simulink library "CPFSK_termpaper"  (R2018a)
settings: Solver=VariableStepAuto  StartTime=0.0  StopTime=10.0  RelTol=1e-3
libraries: dspfdesign x4, commchan3 x1, commrandsrc3 x1, commdigbbndcpm2 x1, simulink x1, dspswit3 x1
settings Model: Creator=Arun Sai  LastModifiedBy=Arun Sai

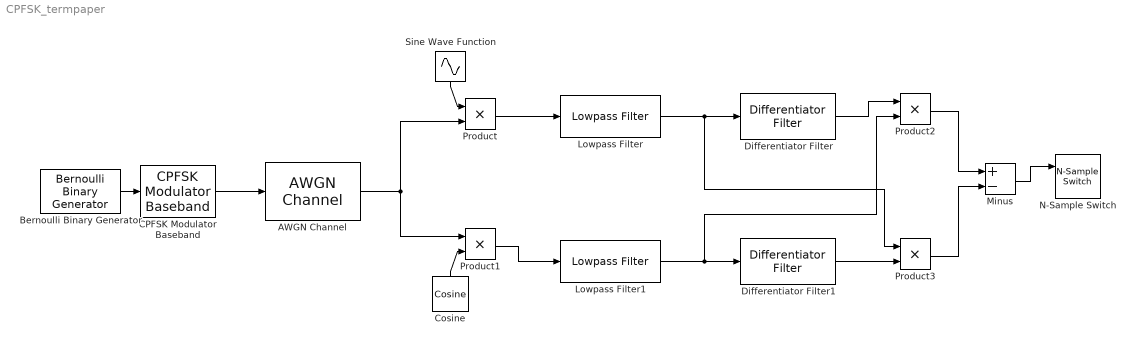
== system CPFSK_termpaper ==
  AWGN Channel : commchan3/AWGN Channel  InputProcessing=Columns as channels (frame based)  seed=67  noiseMode="Signal to noise ratio  (Eb/No)"  EbNodB=10  EsNodB=10  SNRdB=10  bitsPerSym=8  Ps=1  Tsym=1  variance=1
  Bernoulli Binary Generator : commrandsrc3/Bernoulli Binary Generator  ProbabilityOfZero=0.5  SeedSource=Auto  Seed=0  SampleTime=1  SamplesPerFrame=1  OutputDataType=double  SimulateUsing=Interpreted execution
  CPFSK Modulator Baseband : commdigbbndcpm2/CPFSK Modulator Baseband  Mnum=2  inputType=Integer  mappingType=Binary  modIdx=.67  phaseOffset=0  samplesPerSymbol=8  RateOptions=Enforce single-rate processing  outDataType=double
      settings: SourceProductName=Communications System Toolbox  SourceProductBaseCode=CM
  Cosine : simulink/Lookup Tables/Cosine  Formula=cos(2*pi*u)  NumDataPoints=(2^5)+1  OutputWordLength=16  InternalRulePriority=Speed
      settings: SourceProductName=Simulink  SourceProductBaseCode=SL
  Differentiator Filter : dspfdesign/Differentiator Filter  DesignForMinimumOrder=on  FilterOrder=31  PassbandRipple=0.1  ScaleCoefficients=off  SimulateUsing=Interpreted execution  roundingMode=Floor  coeffsDataTypeStr=fixdt(1,16)
      settings: SourceProductName=DSP System Toolbox  SourceProductBaseCode=DS
  Differentiator Filter1 : dspfdesign/Differentiator Filter  DesignForMinimumOrder=on  FilterOrder=31  PassbandRipple=0.1  ScaleCoefficients=off  SimulateUsing=Interpreted execution  roundingMode=Floor  coeffsDataTypeStr=fixdt(1,16)
      settings: SourceProductName=DSP System Toolbox  SourceProductBaseCode=DS
  Lowpass Filter : dspfdesign/Lowpass Filter  FilterType=FIR  DesignForMinimumOrder=on  FilterOrder=50  PassbandFrequency=8e3  StopbandFrequency=12e3  PassbandRipple=0.1  StopbandAttenuation=80  InheritSampleRate=off  SampleRate=44100  SimulateUsing=Interpreted execution  roundingMode=Floor  coeffsDataTypeStr=fixdt(1,16)
  Lowpass Filter1 : dspfdesign/Lowpass Filter  FilterType=FIR  DesignForMinimumOrder=on  FilterOrder=50  PassbandFrequency=8e3  StopbandFrequency=12e3  PassbandRipple=0.1  StopbandAttenuation=80  InheritSampleRate=off  SampleRate=44100  SimulateUsing=Interpreted execution  roundingMode=Floor  coeffsDataTypeStr=fixdt(1,16)
  Minus : Sum  Inputs=+-
  N-Sample Switch : dspswit3/N-Sample Switch  N=8  reset=off  TriggerType=Rising edge  Ts=0.1
      settings: SourceProductName=DSP System Toolbox  SourceProductBaseCode=DS
  Product{,1..3} (4 alike) : Product
  Sine Wave Function : Sin  TimeSource=Use external signal  SampleTime=0
  wires:
  Product/1 -> Lowpass Filter/1
  Sine Wave Function/1 -> Product/1
  Cosine/1 -> Product1/2
  Product1/1 -> Lowpass Filter1/1
  Lowpass Filter/1 -> Differentiator Filter/1, Product3/1
  Lowpass Filter1/1 -> Differentiator Filter1/1, Product2/2
  Differentiator Filter/1 -> Product2/1
  Differentiator Filter1/1 -> Product3/2
  Product2/1 -> Minus/1
  Product3/1 -> Minus/2
  Minus/1 -> N-Sample Switch/1
  AWGN Channel/1 -> Product/2, Product1/1
  CPFSK Modulator Baseband/1 -> AWGN Channel/1
  Bernoulli Binary Generator/1 -> CPFSK Modulator Baseband/1
